simulink model "conSys_3robots_1_vR2014a"  (Simulink 8.3)
settings: Solver=ode3  StartTime=0.0  StopTime=200  FixedStep=Ts  RelTol=1e-3
values from neighbouring files (symbols this model uses):
  ck = double(max(abs([par.q0_r1;par.q0_r2] - [par.q0r_r1;par.q0r_r2]))*20/7000 + 6)    [startUp_conSys_2robots_1_vGPU_vR2014a.m]    (also in startUp_conSys_2robots_1_vR2014a.m = max(abs([par.q0_r1;par.q0_r2] - [par.q0r_r1;par.q0r_r2]))*20; startUp_conSys_2robots_2_vR2014a.m = max(abs([par.q0_r1;par.q0_r2] - [par.q0r_r1;par.q0r_r2]))*20; startUp_conSys_2robots_3_vR2014a.m = max(abs([par.q0_r1;par.q0_r2] - [par.q0r_r1;par.q0r_r2]))*20; startUp_conSys_2robots_4_vR2014a.m = max(abs([par.q0_r1;par.q0_r2] - [par.q0r_r1;par.q0r_r2]))*20)
  d0t = dt*ht    (= 0.328)    [startUp_conSys_2robots_1_vGPU_vR2014a.m]    (also in startUp_conSys_2robots_1_vR2014a.m; startUp_conSys_2robots_2_vR2014a.m; startUp_conSys_2robots_3_vR2014a.m; startUp_conSys_2robots_4_vR2014a.m)
  dt = rt*ht    (= 16.4)    [startUp_conSys_2robots_1_vGPU_vR2014a.m]    (also in startUp_conSys_2robots_1_vR2014a.m; startUp_conSys_2robots_2_vR2014a.m; startUp_conSys_2robots_3_vR2014a.m; startUp_conSys_2robots_4_vR2014a.m)
  dx1r_0 = dxc_0 + sin(thc_0)*dd_0 + d_0*cos(thc_0)*dthc_0    [startUp_conSys_2robots_1_vGPU_vR2014a.m]    (also in startUp_conSys_2robots_1_vR2014a.m; startUp_conSys_2robots_2_vR2014a.m; startUp_conSys_2robots_3_vR2014a.m; startUp_conSys_2robots_4_vR2014a.m)
  dx2r_0 = dxc_0 - sin(thc_0)*dd_0 - d_0*cos(thc_0)*dthc_0    [startUp_conSys_2robots_1_vGPU_vR2014a.m]    (also in startUp_conSys_2robots_1_vR2014a.m; startUp_conSys_2robots_2_vR2014a.m; startUp_conSys_2robots_3_vR2014a.m; startUp_conSys_2robots_4_vR2014a.m)
  dy1r_0 = dyc_0 + cos(thc_0)*dd_0 - d_0*sin(thc_0)*dthc_0    [startUp_conSys_2robots_1_vGPU_vR2014a.m]    (also in startUp_conSys_2robots_1_vR2014a.m; startUp_conSys_2robots_2_vR2014a.m; startUp_conSys_2robots_3_vR2014a.m; startUp_conSys_2robots_4_vR2014a.m)
  dy2r_0 = dyc_0 - cos(thc_0)*dd_0 + d_0*sin(thc_0)*dthc_0    [startUp_conSys_2robots_1_vGPU_vR2014a.m]    (also in startUp_conSys_2robots_1_vR2014a.m; startUp_conSys_2robots_2_vR2014a.m; startUp_conSys_2robots_3_vR2014a.m; startUp_conSys_2robots_4_vR2014a.m)
  ht = .02    (= 0.02)    [startUp_conSys_2robots_1_vGPU_vR2014a.m]    (also in startUp_conSys_2robots_1_vR2014a.m; startUp_conSys_2robots_2_vR2014a.m; startUp_conSys_2robots_3_vR2014a.m; startUp_conSys_2robots_4_vR2014a.m)
  rt = 820    [startUp_conSys_2robots_1_vGPU_vR2014a.m]    (also in startUp_conSys_2robots_1_vR2014a.m; startUp_conSys_2robots_2_vR2014a.m; startUp_conSys_2robots_3_vR2014a.m; startUp_conSys_2robots_4_vR2014a.m)
  TD = ss(Atd,Btd,Ctd,Dtd,Ts)    [startUp_conSys_2robots_1_vGPU_vR2014a.m]    (also in startUp_conSys_2robots_1_vR2014a.m; startUp_conSys_2robots_2_vR2014a.m; startUp_conSys_2robots_3_vR2014a.m; startUp_conSys_2robots_4_vR2014a.m)
  Ts = 1/200    (= 0.005)    [startUp_conSys_2robots_1_vGPU_vR2014a.m]    (also in startUp_conSys_2robots_1_vR2014a.m = 0.0125; startUp_conSys_2robots_2_vR2014a.m = 0.01; startUp_conSys_2robots_3_vR2014a.m; startUp_conSys_2robots_4_vR2014a.m)
undefined symbols (not defined in the file or in its folder): Beta_Correction_1b, Beta_Correction_2b, Beta_Correction_3b, Beta_Correction_4b, DiscIntNeverNeededParam, dth1r_0, dth2r_0, dth3r_0, dx3r_0, dy3r_0, par, th1r_0, th2r_0, th3r_0, x1r_0, x2r_0, x3r_0, y1r_0, y2r_0, y3r_0
undefined symbols (not defined in the file): ADAMS_cwd, ADAMS_exec, ADAMS_host, ADAMS_init, ADAMS_inputs, ADAMS_outputs, ADAMS_prefix, ADAMS_static, ADAMS_sysdir
libraries: simulink x26, cstblocks x11
(part 1 of 3)
settings Model: Creator=baqumau  LastModifiedBy=Mauro
settings DataIOCC: SignalLoggingSaveFormat=Dataset
settings DebuggingCC: UnderspecifiedInitializationDetection=Simplified  StateNameClashWarn=none
settings GRTTargetCC: CombineOutputUpdateFcns=on  GRTInterface=off

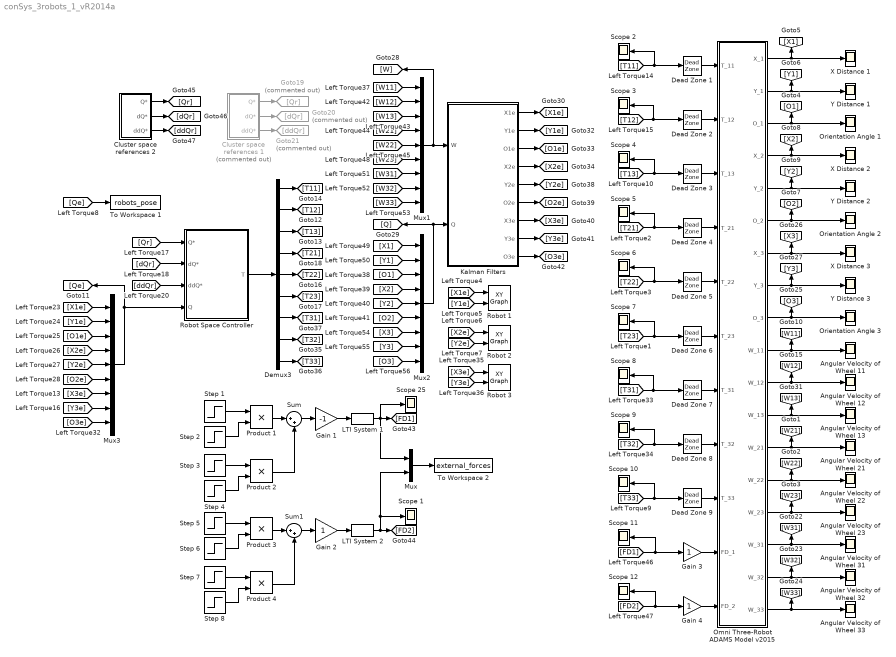
== system conSys_3robots_1_vR2014a ==
  Angular Velocity of Wheel {11..13,21..23,31..33} (9 alike) : Scope
      Angular Velocity of Wheel 11 settings: YMin=-1  YMax=20  SaveName=ScopeData3
      Angular Velocity of Wheel 12 settings: YMin=-1  YMax=1  SaveName=ScopeData2
      Angular Velocity of Wheel 13 settings: YMin=-1  YMax=1  SaveName=ScopeData9
      Angular Velocity of Wheel 21 settings: YMin=-1  YMax=20  SaveName=ScopeData6
      Angular Velocity of Wheel 22 settings: YMin=-1  YMax=1  SaveName=ScopeData10
      Angular Velocity of Wheel 23 settings: YMin=-1  YMax=1  SaveName=ScopeData11
      Angular Velocity of Wheel 31 settings: YMin=-1  YMax=20  SaveName=ScopeData109
      Angular Velocity of Wheel 32 settings: YMin=-1  YMax=1  SaveName=ScopeData110
      Angular Velocity of Wheel 33 settings: YMin=-1  YMax=1  SaveName=ScopeData111
  Cluster space references 1 : Subsystem  Commented=on
  Cluster space references 2 : Subsystem
  Dead Zone {1..9} (9 alike) : DeadZone  LowerValue=-25  UpperValue=25  SaturateOnIntegerOverflow=on
  Demux3 : Demux  Outputs=9
  Gain 1 : Gain  Gain=-1
  Gain 2 : Gain
  Gain 3 : Gain
  Gain 4 : Gain
  Goto19 : Goto  Commented=on  GotoTag=Qr
  Goto20 : Goto  Commented=on  GotoTag=dQr
  Goto21 : Goto  Commented=on  GotoTag=ddQr
  Kalman Filters : Subsystem
  LTI System 1 : cstblocks/LTI System  sys=Fz  IC=[]
  LTI System 2 : cstblocks/LTI System  sys=Fz  IC=[]
  Mux : Mux  Inputs=2
  Mux1 : Mux  Inputs=9
  Mux2 : Mux  Inputs=9
  Mux3 : Mux  Inputs=9
  Omni Three-Robot ADAMS Model v2015 : Subsystem
  Orientation Angle 1 : Scope
      settings: YMin=-3  YMax=3
  Orientation Angle 2 : Scope
      settings: YMin=-3  YMax=3  SaveName=ScopeData12
  Orientation Angle 3 : Scope
      settings: YMin=-3  YMax=3  SaveName=ScopeData112
  Product {1..4} (4 alike) : Product
  Robot 1 : simulink/Sinks/XY Graph  xmin=0  xmax=20000  ymin=0  ymax=20000  st=-1
  Robot 2 : simulink/Sinks/XY Graph  xmin=0  xmax=20000  ymin=0  ymax=20000  st=-1
  Robot 3 : simulink/Sinks/XY Graph  xmin=0  xmax=20000  ymin=0  ymax=20000  st=-1
  Robot Space Controller : Subsystem
  Scope {1..12,25} (13 alike) : Scope
      Scope 1 settings: YMin=-1  YMax=1  SaveName=ScopeData113
      Scope 10 settings: YMin=-6  YMax=6  SaveName=ScopeData124
      Scope 11 settings: YMin=-6  YMax=6  SaveName=ScopeData125
      Scope 12 settings: YMin=-6  YMax=6  SaveName=ScopeData126
      Scope 2 settings: YMin=-6  YMax=6  SaveName=ScopeData114
      Scope 25 settings: YMin=-1  YMax=1  SaveName=ScopeData108
      Scope 3 settings: YMin=-6  YMax=6  SaveName=ScopeData115
      Scope 4 settings: YMin=-6  YMax=6  SaveName=ScopeData116
      Scope 5 settings: YMin=-6  YMax=6  SaveName=ScopeData117
      Scope 6 settings: YMin=-6  YMax=6  SaveName=ScopeData120
      Scope 7 settings: YMin=-6  YMax=6  SaveName=ScopeData121
      Scope 8 settings: YMin=-6  YMax=6  SaveName=ScopeData122
      Scope 9 settings: YMin=-6  YMax=6  SaveName=ScopeData123
  Step 1 : Step  Time=60  SampleTime=0
  Step 2 : Step  Time=100  Before=1  After=0  SampleTime=0
  Step 3 : Step  Time=130  After=-1  SampleTime=0
  Step 4 : Step  Time=170  Before=1  After=0  SampleTime=0
  Step 5 : Step  Time=80  SampleTime=0
  Step 6 : Step  Time=110  Before=1  After=0  SampleTime=0
  Step 7 : Step  Time=120  After=-1  SampleTime=0
  Step 8 : Step  Time=180  Before=1  After=0  SampleTime=0
  Sum : Sum  Inputs=|++
  Sum1 : Sum  Inputs=|++
  To Workspace 1 : ToWorkspace  VariableName=robots_pose  SaveFormat=Structure With Time  SampleTime=-1
  To Workspace 2 : ToWorkspace  VariableName=external_forces  SaveFormat=Structure With Time  SampleTime=-1
  X Distance 1 : Scope
      settings: YMin=0  YMax=10000  SaveName=ScopeData4
  X Distance 2 : Scope
      settings: YMin=0  YMax=10000  SaveName=ScopeData16
  X Distance 3 : Scope
      settings: YMin=0  YMax=10000  SaveName=ScopeData118
  Y Distance 1 : Scope
      settings: YMin=0  YMax=10000
  Y Distance 2 : Scope
      settings: YMin=0  YMax=10000  SaveName=ScopeData17
  Y Distance 3 : Scope
      settings: YMin=3000  YMax=3050  SaveName=ScopeData119
  wires:
  Omni Three-Robot ADAMS Model v2015/1(X_1) -> X Distance 1/1, [X1]
  Omni Three-Robot ADAMS Model v2015/2(Y_1) -> [Y1], Y Distance 1/1
  Omni Three-Robot ADAMS Model v2015/3(O_1) -> [O1], Orientation Angle 1/1
  Omni Three-Robot ADAMS Model v2015/10(W_11) -> [W11], Angular Velocity of Wheel 11/1
  Omni Three-Robot ADAMS Model v2015/11(W_12) -> [W12], Angular Velocity of Wheel 12/1
  Omni Three-Robot ADAMS Model v2015/12(W_13) -> Angular Velocity of Wheel 13/1, [W13]
  Omni Three-Robot ADAMS Model v2015/4(X_2) -> X Distance 2/1, [X2]
  Omni Three-Robot ADAMS Model v2015/5(Y_2) -> Y Distance 2/1, [Y2]
  Omni Three-Robot ADAMS Model v2015/6(O_2) -> Orientation Angle 2/1, [O2]
  Omni Three-Robot ADAMS Model v2015/13(W_21) -> Angular Velocity of Wheel 21/1, [W21]
  Omni Three-Robot ADAMS Model v2015/14(W_22) -> Angular Velocity of Wheel 22/1, [W22]
  Omni Three-Robot ADAMS Model v2015/15(W_23) -> [W23], Angular Velocity of Wheel 23/1
  [X1e] -> Robot 1/1
  [Y1e] -> Robot 1/2
  [X2e] -> Robot 2/1
  [Y2e] -> Robot 2/2
  [O1e] -> Mux3/3
  [X2e] -> Mux3/4
  [Y2e] -> Mux3/5
  [O2e] -> Mux3/6
  [X1e] -> Mux3/1
  [Y1e] -> Mux3/2
  [Qr] -> Robot Space Controller/1(Q*)
  [dQr] -> Robot Space Controller/2(dQ*)
  Mux3/1 -> Robot Space Controller/4(Q), [Qe]
  Robot Space Controller/1(T) -> Demux3/1
  Demux3/1 -> [T11]
  Demux3/2 -> [T12]
  Demux3/3 -> [T13]
  Demux3/4 -> [T21]
  Demux3/5 -> [T22]
  Demux3/6 -> [T23]
  [ddQr] -> Robot Space Controller/3(ddQ*)
  Omni Three-Robot ADAMS Model v2015/7(X_3) -> [X3], X Distance 3/1
  Omni Three-Robot ADAMS Model v2015/8(Y_3) -> [Y3], Y Distance 3/1
  Omni Three-Robot ADAMS Model v2015/9(O_3) -> [O3], Orientation Angle 3/1
  Omni Three-Robot ADAMS Model v2015/16(W_31) -> [W31], Angular Velocity of Wheel 31/1
  Omni Three-Robot ADAMS Model v2015/17(W_32) -> [W32], Angular Velocity of Wheel 32/1
  Omni Three-Robot ADAMS Model v2015/18(W_33) -> Angular Velocity of Wheel 33/1, [W33]
  [X3e] -> Robot 3/1
  [Y3e] -> Robot 3/2
  Cluster space references 1/1(Q*) -> Goto19/1
  Cluster space references 1/2(dQ*) -> Goto20/1
  Cluster space references 1/3(ddQ*) -> Goto21/1
  [X3e] -> Mux3/7
  [Y3e] -> Mux3/8
  [O3e] -> Mux3/9
  Demux3/7 -> [T31]
  Demux3/8 -> [T32]
  Demux3/9 -> [T33]
  [FD2] -> Gain 4/1, Scope 12/1
  [FD1] -> Gain 3/1, Scope 11/1
  [T13] -> Dead Zone 3/1, Scope 4/1
  [T22] -> Dead Zone 5/1, Scope 6/1
  [T31] -> Dead Zone 7/1, Scope 8/1
  [T33] -> Dead Zone 9/1, Scope 10/1
  [T23] -> Dead Zone 6/1, Scope 7/1
  [T12] -> Dead Zone 2/1, Scope 3/1
  [T11] -> Dead Zone 1/1, Scope 2/1
  [T32] -> Dead Zone 8/1, Scope 9/1
  [T21] -> Dead Zone 4/1, Scope 5/1
  [W13] -> Mux1/3
  [W21] -> Mux1/4
  [W22] -> Mux1/5
  [W23] -> Mux1/6
  [W11] -> Mux1/1
  [W12] -> Mux1/2
  Mux1/1 -> [W], Kalman Filters/1(W)
  [O1] -> Mux2/3
  [X2] -> Mux2/4
  [Y2] -> Mux2/5
  [O2] -> Mux2/6
  [X1] -> Mux2/1
  [Y1] -> Mux2/2
  Mux2/1 -> Kalman Filters/2(Q), [Q]
  Kalman Filters/1(X1e) -> [X1e]
  Kalman Filters/2(Y1e) -> [Y1e]
  Kalman Filters/3(O1e) -> [O1e]
  Kalman Filters/4(X2e) -> [X2e]
  Kalman Filters/5(Y2e) -> [Y2e]
  Kalman Filters/6(O2e) -> [O2e]
  [W31] -> Mux1/7
  [W32] -> Mux1/8
  [W33] -> Mux1/9
  [X3] -> Mux2/7
  [Y3] -> Mux2/8
  [O3] -> Mux2/9
  Kalman Filters/7(X3e) -> [X3e]
  Kalman Filters/8(Y3e) -> [Y3e]
  Kalman Filters/9(O3e) -> [O3e]
  [Qe] -> To Workspace 1/1
  Step 1/1 -> Product 1/1
  Step 2/1 -> Product 1/2
  Step 3/1 -> Product 2/1
  Step 4/1 -> Product 2/2
  Product 1/1 -> Sum/1
  Product 2/1 -> Sum/2
  Sum/1 -> Gain 1/1
  Gain 1/1 -> LTI System 1/1
  Step 5/1 -> Product 3/1
  Step 6/1 -> Product 3/2
  Step 7/1 -> Product 4/1
  Step 8/1 -> Product 4/2
  Product 3/1 -> Sum1/1
  Product 4/1 -> Sum1/2
  Sum1/1 -> Gain 2/1
  LTI System 2/1 -> [FD2], Mux/2, Scope 1/1
  Gain 2/1 -> LTI System 2/1
  LTI System 1/1 -> Mux/1, Scope 25/1, [FD1]
  Mux/1 -> To Workspace 2/1
  Cluster space references 2/1(Q*) -> [Qr]
  Cluster space references 2/2(dQ*) -> [dQr]
  Cluster space references 2/3(ddQ*) -> [ddQr]
  Dead Zone 1/1 -> Omni Three-Robot ADAMS Model v2015/1(T_11)
  Dead Zone 2/1 -> Omni Three-Robot ADAMS Model v2015/2(T_12)
  Dead Zone 3/1 -> Omni Three-Robot ADAMS Model v2015/3(T_13)
  Dead Zone 4/1 -> Omni Three-Robot ADAMS Model v2015/4(T_21)
  Dead Zone 5/1 -> Omni Three-Robot ADAMS Model v2015/5(T_22)
  Dead Zone 6/1 -> Omni Three-Robot ADAMS Model v2015/6(T_23)
  Dead Zone 7/1 -> Omni Three-Robot ADAMS Model v2015/7(T_31)
  Dead Zone 8/1 -> Omni Three-Robot ADAMS Model v2015/8(T_32)
  Dead Zone 9/1 -> Omni Three-Robot ADAMS Model v2015/9(T_33)
  Gain 3/1 -> Omni Three-Robot ADAMS Model v2015/10(FD_1)
  Gain 4/1 -> Omni Three-Robot ADAMS Model v2015/11(FD_2)

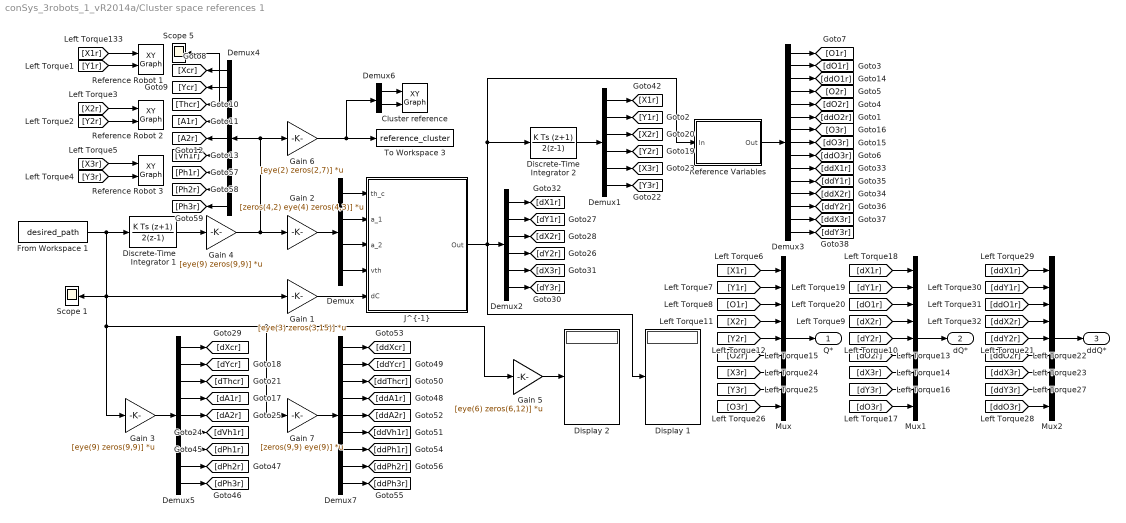
== system conSys_3robots_1_vR2014a/Cluster space references 1 ==
  Cluster reference : simulink/Sinks/XY Graph  xmin=0  xmax=20000  ymin=0  ymax=20000  st=-1
  Demux : Demux
  Demux1 : Demux  Outputs=6
  Demux2 : Demux  Outputs=6
  Demux3 : Demux  Outputs=15
  Demux4 : Demux  Outputs=9
  Demux5 : Demux  Outputs=9
  Demux6 : Demux  Outputs=2
  Demux7 : Demux  Outputs=9
  Discrete-Time Integrator 1 : DiscreteIntegrator  IntegratorMethod=Integration: Trapezoidal  InitialCondition=par.x0_c_ref  SampleTime=Ts  ICPrevOutput=DiscIntNeverNeededParam  ICPrevScaledInput=DiscIntNeverNeededParam
  Discrete-Time Integrator 2 : DiscreteIntegrator  IntegratorMethod=Integration: Trapezoidal  InitialCondition=[x1r_0 y1r_0 x2r_0 y2r_0 x3r_0 y3r_0]'  SampleTime=Ts  ICPrevOutput=DiscIntNeverNeededParam  ICPrevScaledInput=DiscIntNeverNeededParam
  Display 1 : Display
  Display 2 : Display
  From Workspace 1 : FromWorkspace  VariableName=desired_path  SampleTime=Ts  OutputAfterFinalValue=Holding final value
  Gain 1 : Gain  Gain=[eye(3) zeros(3,15)]  Multiplication=Matrix(K*u)
  Gain 2 : Gain  Gain=[zeros(4,2) eye(4) zeros(4,3)]  Multiplication=Matrix(K*u)
  Gain 3 : Gain  Gain=[eye(9) zeros(9,9)]  Multiplication=Matrix(K*u)
  Gain 4 : Gain  Gain=[eye(9) zeros(9,9)]  Multiplication=Matrix(K*u)
  Gain 5 : Gain  Gain=[eye(6) zeros(6,12)]  Multiplication=Matrix(K*u)
  Gain 6 : Gain  Gain=[eye(2) zeros(2,7)]  Multiplication=Matrix(K*u)
  Gain 7 : Gain  Gain=[zeros(9,9) eye(9)]  Multiplication=Matrix(K*u)
  "J^{-1}" : Subsystem
  Mux : Mux  Inputs=9
  Mux1 : Mux  Inputs=9
  Mux2 : Mux  Inputs=9
  Reference Robot 1 : simulink/Sinks/XY Graph  xmin=0  xmax=20000  ymin=0  ymax=20000  st=-1
  Reference Robot 2 : simulink/Sinks/XY Graph  xmin=0  xmax=20000  ymin=0  ymax=20000  st=-1
  Reference Robot 3 : simulink/Sinks/XY Graph  xmin=0  xmax=20000  ymin=0  ymax=20000  st=-1
  Reference Variables : Subsystem
  Scope 1 : Scope
      settings: ShowLegends=on  YMin=-500  YMax=500  SaveName=ScopeData32
  Scope 5 : Scope
      settings: ShowLegends=on  YMin=-500  YMax=500  SaveName=ScopeData100
  To Workspace 3 : ToWorkspace  VariableName=reference_cluster  SaveFormat=Structure With Time  SampleTime=-1
  Q* : Outport
  dQ* : Outport  Port=2
  ddQ* : Outport  Port=3
  wires:
  From Workspace 1/1 -> Scope 1/1, Gain 3/1, Gain 7/1, Gain 5/1, Gain 1/1, Discrete-Time Integrator 1/1
  Discrete-Time Integrator 1/1 -> Gain 4/1
  "J^{-1}"/1(Out) -> Display 1/1, Demux2/1, Reference Variables/1(In), Discrete-Time Integrator 2/1
  Discrete-Time Integrator 2/1 -> Demux1/1
  Demux1/1 -> [X1r]
  Demux1/2 -> [Y1r]
  [X1r] -> Reference Robot 1/1
  [Y1r] -> Reference Robot 1/2
  [X2r] -> Reference Robot 2/1
  [Y2r] -> Reference Robot 2/2
  [X3r] -> Reference Robot 3/1
  [Y3r] -> Reference Robot 3/2
  Demux2/1 -> [dX1r]
  Demux2/2 -> [dY1r]
  Demux2/5 -> [dX3r]
  Demux2/6 -> [dY3r]
  Gain 6/1 -> To Workspace 3/1, Demux6/1
  Demux/2 -> "J^{-1}"/2(a_1)
  Demux/3 -> "J^{-1}"/3(a_2)
  Demux/4 -> "J^{-1}"/4(vth)
  Demux/1 -> "J^{-1}"/1(th_c)
  Gain 1/1 -> "J^{-1}"/5(dC)
  Demux2/3 -> [dX2r]
  Demux2/4 -> [dY2r]
  Demux1/3 -> [X2r]
  Demux1/4 -> [Y2r]
  Demux1/5 -> [X3r]
  Demux1/6 -> [Y3r]
  Reference Variables/1(Out) -> Demux3/1
  Demux3/1 -> [O1r]
  Demux3/2 -> [dO1r]
  Gain 2/1 -> Demux/1
  [X2r] -> Mux/4
  [O1r] -> Mux/3
  [Y1r] -> Mux/2
  [Y2r] -> Mux/5
  [X1r] -> Mux/1
  [O2r] -> Mux/6
  Mux/1 -> Q*/1
  Mux1/1 -> dQ*/1
  Demux4/1 -> [Xcr]
  Demux4/2 -> [Ycr]
  Demux4/3 -> Scope 5/1, [Thcr]
  Demux4/4 -> [A1r]
  Demux4/5 -> [A2r]
  Demux4/6 -> [Vh1r]
  [Y3r] -> Mux/8
  [X3r] -> Mux/7
  [O3r] -> Mux/9
  Demux5/1 -> [dXcr]
  Demux5/2 -> [dYcr]
  Demux5/3 -> [dThcr]
  Demux5/4 -> [dA1r]
  Demux5/5 -> [dA2r]
  Demux5/6 -> [dVh1r]
  Demux6/2 -> Cluster reference/2
  Demux6/1 -> Cluster reference/1
  Gain 3/1 -> Demux5/1
  Gain 4/1 -> Demux4/1, Gain 6/1, Gain 2/1
  Gain 5/1 -> Display 2/1
  Demux5/7 -> [dPh1r]
  Demux5/8 -> [dPh2r]
  Demux5/9 -> [dPh3r]
  Demux7/1 -> [ddXcr]
  Demux7/2 -> [ddYcr]
  Demux7/3 -> [ddThcr]
  Demux7/4 -> [ddA1r]
  Demux7/5 -> [ddA2r]
  Demux7/6 -> [ddVh1r]
  Gain 7/1 -> Demux7/1
  Demux7/7 -> [ddPh1r]
  Demux7/8 -> [ddPh2r]
  Demux7/9 -> [ddPh3r]
  Demux4/7 -> [Ph1r]
  Demux4/8 -> [Ph2r]
  Demux4/9 -> [Ph3r]
  Mux2/1 -> ddQ*/1
  [ddX2r] -> Mux2/4
  [ddO1r] -> Mux2/3
  [ddY1r] -> Mux2/2
  [ddY2r] -> Mux2/5
  [ddX1r] -> Mux2/1
  [ddO2r] -> Mux2/6
  [ddY3r] -> Mux2/8
  [ddX3r] -> Mux2/7
  [ddO3r] -> Mux2/9
  [dX2r] -> Mux1/4
  [dO1r] -> Mux1/3
  [dY1r] -> Mux1/2
  [dY2r] -> Mux1/5
  [dX1r] -> Mux1/1
  [dO2r] -> Mux1/6
  [dY3r] -> Mux1/8
  [dX3r] -> Mux1/7
  [dO3r] -> Mux1/9
  Demux3/3 -> [ddO1r]
  Demux3/4 -> [O2r]
  Demux3/5 -> [dO2r]
  Demux3/6 -> [ddO2r]
  Demux3/7 -> [O3r]
  Demux3/8 -> [dO3r]
  Demux3/9 -> [ddO3r]
  Demux3/10 -> [ddX1r]
  Demux3/11 -> [ddY1r]
  Demux3/12 -> [ddX2r]
  Demux3/13 -> [ddY2r]
  Demux3/14 -> [ddX3r]
  Demux3/15 -> [ddY3r]

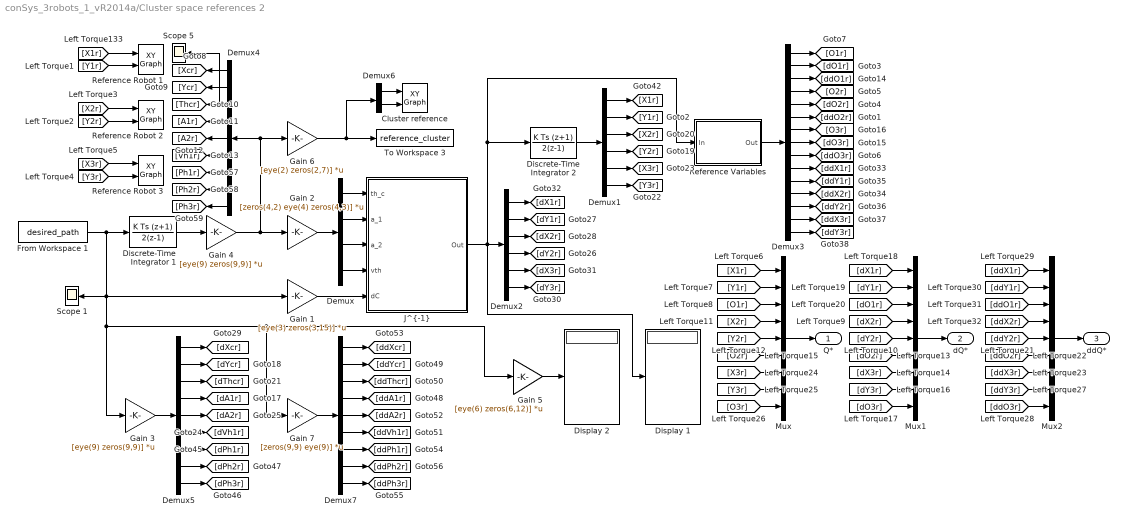
== system conSys_3robots_1_vR2014a/Cluster space references 2 ==
  Cluster reference : simulink/Sinks/XY Graph  xmin=0  xmax=20000  ymin=0  ymax=20000  st=-1
  Demux : Demux
  Demux1 : Demux  Outputs=6
  Demux2 : Demux  Outputs=6
  Demux3 : Demux  Outputs=15
  Demux4 : Demux  Outputs=9
  Demux5 : Demux  Outputs=9
  Demux6 : Demux  Outputs=2
  Demux7 : Demux  Outputs=9
  Discrete-Time Integrator 1 : DiscreteIntegrator  IntegratorMethod=Integration: Trapezoidal  InitialCondition=par.x0_c_ref  SampleTime=Ts  ICPrevOutput=DiscIntNeverNeededParam  ICPrevScaledInput=DiscIntNeverNeededParam
  Discrete-Time Integrator 2 : DiscreteIntegrator  IntegratorMethod=Integration: Trapezoidal  InitialCondition=[x1r_0 y1r_0 x2r_0 y2r_0 x3r_0 y3r_0]'  SampleTime=Ts  ICPrevOutput=DiscIntNeverNeededParam  ICPrevScaledInput=DiscIntNeverNeededParam
  Display 1 : Display
  Display 2 : Display
  From Workspace 1 : FromWorkspace  VariableName=desired_path  SampleTime=Ts  OutputAfterFinalValue=Holding final value
  Gain 1 : Gain  Gain=[eye(3) zeros(3,15)]  Multiplication=Matrix(K*u)
  Gain 2 : Gain  Gain=[zeros(4,2) eye(4) zeros(4,3)]  Multiplication=Matrix(K*u)
  Gain 3 : Gain  Gain=[eye(9) zeros(9,9)]  Multiplication=Matrix(K*u)
  Gain 4 : Gain  Gain=[eye(9) zeros(9,9)]  Multiplication=Matrix(K*u)
  Gain 5 : Gain  Gain=[eye(6) zeros(6,12)]  Multiplication=Matrix(K*u)
  Gain 6 : Gain  Gain=[eye(2) zeros(2,7)]  Multiplication=Matrix(K*u)
  Gain 7 : Gain  Gain=[zeros(9,9) eye(9)]  Multiplication=Matrix(K*u)
  "J^{-1}" : Subsystem
  Mux : Mux  Inputs=9
  Mux1 : Mux  Inputs=9
  Mux2 : Mux  Inputs=9
  Reference Robot 1 : simulink/Sinks/XY Graph  xmin=0  xmax=20000  ymin=0  ymax=20000  st=-1
  Reference Robot 2 : simulink/Sinks/XY Graph  xmin=0  xmax=20000  ymin=0  ymax=20000  st=-1
  Reference Robot 3 : simulink/Sinks/XY Graph  xmin=0  xmax=20000  ymin=0  ymax=20000  st=-1
  Reference Variables : Subsystem
  Scope 1 : Scope
      settings: ShowLegends=on  YMin=-500  YMax=500  SaveName=ScopeData32
  Scope 5 : Scope
      settings: ShowLegends=on  YMin=-500  YMax=500  SaveName=ScopeData100
  To Workspace 3 : ToWorkspace  VariableName=reference_cluster  SaveFormat=Structure With Time  SampleTime=-1
  Q* : Outport
  dQ* : Outport  Port=2
  ddQ* : Outport  Port=3
  wires:
  Demux3/15 -> [ddY3r]
  Demux3/14 -> [ddX3r]
  Demux3/13 -> [ddY2r]
  Demux3/12 -> [ddX2r]
  Demux3/11 -> [ddY1r]
  Demux3/10 -> [ddX1r]
  Demux3/9 -> [ddO3r]
  Demux3/8 -> [dO3r]
  Demux3/7 -> [O3r]
  Demux3/6 -> [ddO2r]
  Demux3/5 -> [dO2r]
  Demux3/4 -> [O2r]
  Demux3/3 -> [ddO1r]
  [dO3r] -> Mux1/9
  [dX3r] -> Mux1/7
  [dY3r] -> Mux1/8
  [dO2r] -> Mux1/6
  [dX1r] -> Mux1/1
  [dY2r] -> Mux1/5
  [dY1r] -> Mux1/2
  [dO1r] -> Mux1/3
  [dX2r] -> Mux1/4
  [ddO3r] -> Mux2/9
  [ddX3r] -> Mux2/7
  [ddY3r] -> Mux2/8
  [ddO2r] -> Mux2/6
  [ddX1r] -> Mux2/1
  [ddY2r] -> Mux2/5
  [ddY1r] -> Mux2/2
  [ddO1r] -> Mux2/3
  [ddX2r] -> Mux2/4
  Mux2/1 -> ddQ*/1
  Demux4/9 -> [Ph3r]
  Demux4/8 -> [Ph2r]
  Demux4/7 -> [Ph1r]
  Demux7/9 -> [ddPh3r]
  Demux7/8 -> [ddPh2r]
  Demux7/7 -> [ddPh1r]
  Gain 7/1 -> Demux7/1
  Demux7/6 -> [ddVh1r]
  Demux7/5 -> [ddA2r]
  Demux7/4 -> [ddA1r]
  Demux7/3 -> [ddThcr]
  Demux7/2 -> [ddYcr]
  Demux7/1 -> [ddXcr]
  Demux5/9 -> [dPh3r]
  Demux5/8 -> [dPh2r]
  Demux5/7 -> [dPh1r]
  Gain 5/1 -> Display 2/1
  Gain 4/1 -> Gain 2/1, Gain 6/1, Demux4/1
  Gain 3/1 -> Demux5/1
  Demux6/1 -> Cluster reference/1
  Demux6/2 -> Cluster reference/2
  Demux5/6 -> [dVh1r]
  Demux5/5 -> [dA2r]
  Demux5/4 -> [dA1r]
  Demux5/3 -> [dThcr]
  Demux5/2 -> [dYcr]
  Demux5/1 -> [dXcr]
  [O3r] -> Mux/9
  [X3r] -> Mux/7
  [Y3r] -> Mux/8
  Demux4/6 -> [Vh1r]
  Demux4/5 -> [A2r]
  Demux4/4 -> [A1r]
  Demux4/3 -> [Thcr], Scope 5/1
  Demux4/2 -> [Ycr]
  Demux4/1 -> [Xcr]
  Mux1/1 -> dQ*/1
  Mux/1 -> Q*/1
  [O2r] -> Mux/6
  [X1r] -> Mux/1
  [Y2r] -> Mux/5
  [Y1r] -> Mux/2
  [O1r] -> Mux/3
  [X2r] -> Mux/4
  Gain 2/1 -> Demux/1
  Demux3/2 -> [dO1r]
  Demux3/1 -> [O1r]
  Reference Variables/1(Out) -> Demux3/1
  Demux1/6 -> [Y3r]
  Demux1/5 -> [X3r]
  Demux1/4 -> [Y2r]
  Demux1/3 -> [X2r]
  Demux2/4 -> [dY2r]
  Demux2/3 -> [dX2r]
  Gain 1/1 -> "J^{-1}"/5(dC)
  Demux/1 -> "J^{-1}"/1(th_c)
  Demux/4 -> "J^{-1}"/4(vth)
  Demux/3 -> "J^{-1}"/3(a_2)
  Demux/2 -> "J^{-1}"/2(a_1)
  Gain 6/1 -> Demux6/1, To Workspace 3/1
  Demux2/6 -> [dY3r]
  Demux2/5 -> [dX3r]
  Demux2/2 -> [dY1r]
  Demux2/1 -> [dX1r]
  [Y3r] -> Reference Robot 3/2
  [X3r] -> Reference Robot 3/1
  [Y2r] -> Reference Robot 2/2
  [X2r] -> Reference Robot 2/1
  [Y1r] -> Reference Robot 1/2
  [X1r] -> Reference Robot 1/1
  Demux1/2 -> [Y1r]
  Demux1/1 -> [X1r]
  Discrete-Time Integrator 2/1 -> Demux1/1
  "J^{-1}"/1(Out) -> Discrete-Time Integrator 2/1, Reference Variables/1(In), Demux2/1, Display 1/1
  Discrete-Time Integrator 1/1 -> Gain 4/1
  From Workspace 1/1 -> Discrete-Time Integrator 1/1, Gain 1/1, Gain 5/1, Gain 7/1, Gain 3/1, Scope 1/1

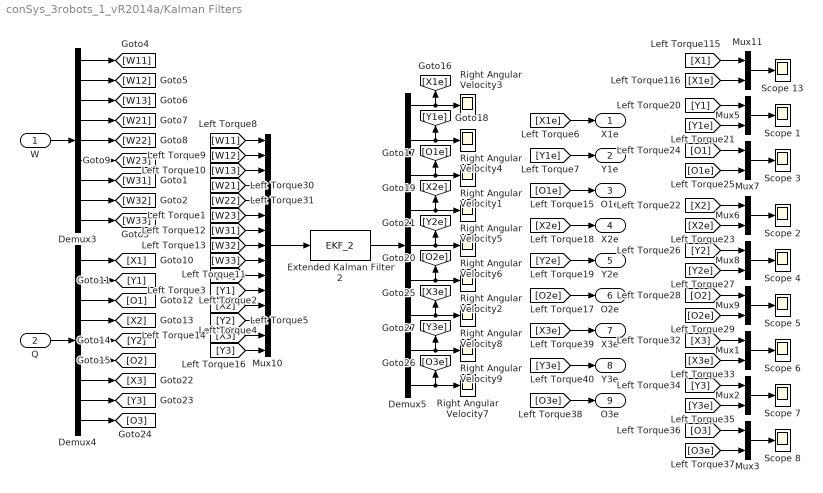
== system conSys_3robots_1_vR2014a/Kalman Filters ==
  W : Inport
  Q : Inport  Port=2
  Demux3 : Demux  Outputs=9
  Demux4 : Demux  Outputs=9
  Demux5 : Demux  Outputs=9
  Extended Kalman Filter 2 : S-Function  FunctionName=EKF_2  Parameters=par  EnableBusSupport=off
  Mux{1..3,5..9,11} (9 alike) : Mux  Inputs=2
  Mux10 : Mux  Inputs=15
  Right Angular Velocity{1..9} (9 alike) : Scope
      Right Angular Velocity1 settings: YMin=-3  YMax=6  SaveName=ScopeData5
      Right Angular Velocity2 settings: YMin=-3  YMax=6  SaveName=ScopeData13
      Right Angular Velocity3 settings: YMin=-10000  YMax=10000  SaveName=ScopeData7
      Right Angular Velocity4 settings: YMin=0  YMax=5000  SaveName=ScopeData8
      Right Angular Velocity5 settings: YMin=-10000  YMax=10000  SaveName=ScopeData14
      Right Angular Velocity6 settings: YMin=0  YMax=5000  SaveName=ScopeData15
      Right Angular Velocity7 settings: YMin=-3  YMax=6  SaveName=ScopeData18
      Right Angular Velocity8 settings: YMin=-10000  YMax=10000  SaveName=ScopeData19
      Right Angular Velocity9 settings: YMin=0  YMax=5000  SaveName=ScopeData20
  Scope {1..8,13} (9 alike) : Scope
      Scope 1 settings: YMin=0  YMax=20000  SaveName=ScopeData29
      Scope 13 settings: YMin=0  YMax=20000  SaveName=ScopeData25
      Scope 2 settings: YMin=-2  YMax=20000  SaveName=ScopeData32
      Scope 3 settings: YMin=-20  YMax=20  SaveName=ScopeData33
      Scope 4 settings: YMin=-2  YMax=20000  SaveName=ScopeData34
      Scope 5 settings: YMin=-20  YMax=20  SaveName=ScopeData35
      Scope 6 settings: YMin=-2  YMax=20000  SaveName=ScopeData21
      Scope 7 settings: YMin=-2  YMax=20000  SaveName=ScopeData23
      Scope 8 settings: YMin=-20  YMax=20  SaveName=ScopeData24
  X1e : Outport
  Y1e : Outport  Port=2
  O1e : Outport  Port=3
  X2e : Outport  Port=4
  Y2e : Outport  Port=5
  O2e : Outport  Port=6
  X3e : Outport  Port=7
  Y3e : Outport  Port=8
  O3e : Outport  Port=9
  wires:
  W/1 -> Demux3/1
  Demux3/1 -> [W11]
  Demux3/2 -> [W12]
  Demux3/3 -> [W13]
  Demux3/4 -> [W21]
  Demux3/5 -> [W22]
  Demux3/6 -> [W23]
  Demux4/1 -> [X1]
  Demux4/2 -> [Y1]
  Demux4/3 -> [O1]
  Demux4/4 -> [X2]
  Demux4/5 -> [Y2]
  Demux4/6 -> [O2]
  Q/1 -> Demux4/1
  [X1e] -> X1e/1
  [Y1e] -> Y1e/1
  [O1e] -> O1e/1
  [X2e] -> X2e/1
  [Y2e] -> Y2e/1
  [O2e] -> O2e/1
  [X1e] -> Mux11/2
  Mux11/1 -> Scope 13/1
  [X1] -> Mux11/1
  [Y1e] -> Mux5/2
  Mux5/1 -> Scope 1/1
  [Y1] -> Mux5/1
  [X2e] -> Mux6/2
  Mux6/1 -> Scope 2/1
  [X2] -> Mux6/1
  [O1e] -> Mux7/2
  Mux7/1 -> Scope 3/1
  [O1] -> Mux7/1
  [Y2e] -> Mux8/2
  Mux8/1 -> Scope 4/1
  [Y2] -> Mux8/1
  [O2e] -> Mux9/2
  Mux9/1 -> Scope 5/1
  [O2] -> Mux9/1
  [W11] -> Mux10/1
  [W12] -> Mux10/2
  [W13] -> Mux10/3
  Mux10/1 -> Extended Kalman Filter 2/1
  Extended Kalman Filter 2/1 -> Demux5/1
  Demux5/2 -> Right Angular Velocity4/1, [Y1e]
  Demux5/3 -> Right Angular Velocity1/1, [O1e]
  Demux5/1 -> Right Angular Velocity3/1, [X1e]
  [W21] -> Mux10/4
  [W22] -> Mux10/5
  Demux5/5 -> [Y2e], Right Angular Velocity6/1
  Demux5/6 -> [O2e], Right Angular Velocity2/1
  Demux5/4 -> [X2e], Right Angular Velocity5/1
  [W23] -> Mux10/6
  Demux3/7 -> [W31]
  Demux3/8 -> [W32]
  Demux3/9 -> [W33]
  Demux4/7 -> [X3]
  Demux4/8 -> [Y3]
  Demux4/9 -> [O3]
  [X2] -> Mux10/12
  [X1] -> Mux10/10
  [Y1] -> Mux10/11
  [Y2] -> Mux10/13
  [X3] -> Mux10/14
  [W31] -> Mux10/7
  [Y3] -> Mux10/15
  [W32] -> Mux10/8
  [W33] -> Mux10/9
  Demux5/8 -> Right Angular Velocity9/1, [Y3e]
  Demux5/9 -> Right Angular Velocity7/1, [O3e]
  Demux5/7 -> Right Angular Velocity8/1, [X3e]
  [X3e] -> Mux1/2
  Mux1/1 -> Scope 6/1
  [X3] -> Mux1/1
  [Y3e] -> Mux2/2
  Mux2/1 -> Scope 7/1
  [Y3] -> Mux2/1
  [O3e] -> Mux3/2
  Mux3/1 -> Scope 8/1
  [O3] -> Mux3/1
  [X3e] -> X3e/1
  [Y3e] -> Y3e/1
  [O3e] -> O3e/1

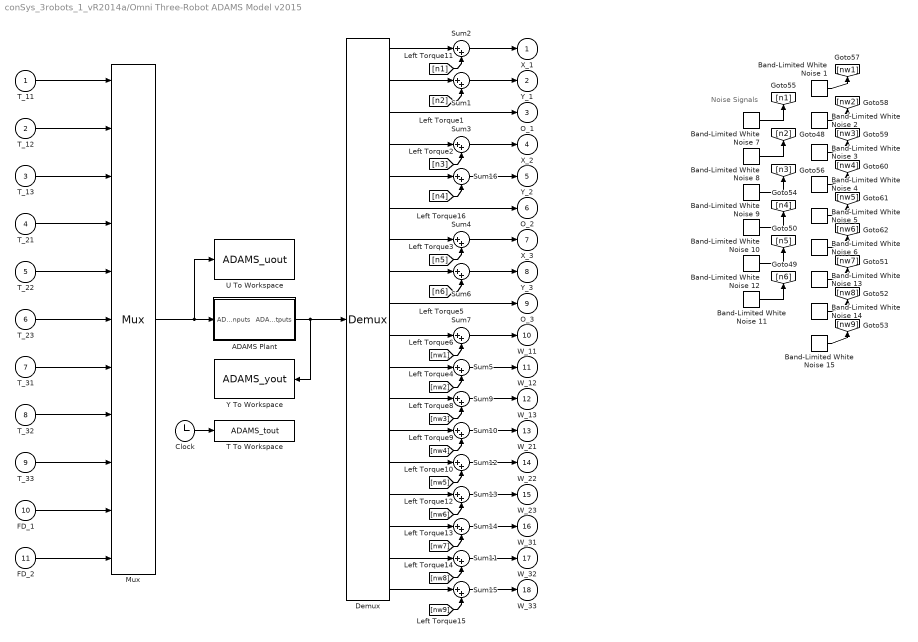
== system conSys_3robots_1_vR2014a/Omni Three-Robot ADAMS Model v2015 ==
  note: Noise Signals
  T_11 : Inport
  T_12 : Inport  Port=2
  T_13 : Inport  Port=3
  T_21 : Inport  Port=4
  T_22 : Inport  Port=5
  T_23 : Inport  Port=6
  T_31 : Inport  Port=7
  T_32 : Inport  Port=8
  T_33 : Inport  Port=9
  FD_1 : Inport  Port=10
  FD_2 : Inport  Port=11
  ADAMS Plant : Subsystem  LoadFcn=|  InitFcn=clear mex  mask(Adams Plant){exevie=ADAMS_sysdir, nam_in=ADAMS_inputs, namout=ADAMS_outputs, nampre=ADAMS_prefix, outfil=ADAMS_prefix, exesol=ADAMS_exec, stat=ADAMS_static, inicmd=[ADAMS_init], exetyp=C++, comtyp=PIPE(DDE), workdir=ADAMS_cwd, ada_host=ADAMS_host, modani=batch, modsim=discrete, dft=no, simulink_lead_cosim=yes, pin_interp_order=0, pout_extrap_order=0, pin_extrap_order=0, pout_interp_order=0, dt_out=Ts, o_rate=1, more=off}
      | %check based on dialog box setting for when setting by popup menu                                             
      | if exist('ADAMS_solver_type')                                                                                 
      |   if strcmp(ADAMS_solver_type,'C++')                                                                          
      |     set_param(gcb,'exetyp','C++');                                                                            
      |   else                                                                                                        
      |     set_param(gcb,'exetyp','Fortran');                                                                        
      |   end                                                                                                         
      | else                                                                                                          
      |   set_param(gcb,'exetyp','C++');                                                                              
      | end                                                                                                           
      | %set the mode if using acar_solver                                                                            
      | %REQUIRED HERE BECAUSE BELOW CAUSES MDLTERMINATE TO BE CALLED 2 TIMES IN MIDDLE OF SIMULATION WHEN SET IN MASK
      |                                                                                                               
      | %enable the direct feedthrough, sim mode, anim mode parameters by default                                     
      |                                                                                                               
      | if exist('set_some_params_states')                                                                            
      |                                                                                                               
      |   set_some_params_states({'dft','modsim','modani'},{'on','on','on'},'MaskEnables',gcb)                        
      |   %turn on direct feedthrough option                                                                          
      |   set_some_params_states({'dft'},{'on'},'MaskVisibilities',gcb)                                               
      |                                                                                                               
      |  end                                                                                                          
      |                                                                                                               
      |                                                                                                               
      | if exist('ADAMS_exec')                                                                                        
      |   if and(strcmp(get_param(gcb,'exesol'),'ADAMS_exec'),strcmp(ADAMS_exec,'acar_solver'))                       
      |     %set the sim mode to discrete -- only supported mode                                                      
      |     set_param(gcb,'modsim','discrete')                                                                        
      |      %turn off direct feedthrough option                                                                      
      |      set_some_params_states({'dft'},{'off'},'MaskVisibilities',gcb)                                           
      |     %set the animation mode to batch -- only supported mode                                                   
      |     set_param(gcb,'modani','batch')                                                                           
      |     %disable the direct feedthrough, sim mode, anim mode parameters                                           
      |     set_some_params_states({'modsim','modani'},{'off','off'},'MaskEnables',gcb)                               
      |   end                                                                                                         
      | end
      mask prompts: exevie "Adams install directory"; nam_in "Adams/View input names"; namout "Adams/View output names"; nampre "Adams model file prefix"; outfil "Output files prefix (opt.: if blank - no output)"; exesol "User executable (opt.: if blank - use standard)"; stat "Initial static simulation flag"; inicmd "Initialization commands"; exetyp "Adams/Solver type"; comtyp "Interprocess option"; workdir "Adams working directory"; ada_host "Adams host"; modani "Animation mode"; modsim "Simulation mode"; dft "Direct feedthrough"; simulink_lead_cosim "Discrete Computational Order - Simulink Leads Adams"; pin_interp_order "Plant input interpolation order"; pout_extrap_order "Plant output extrapolation order"; pin_extrap_order "Plant input extrapolation order"; pout_interp_order "Plant output interpolation order"; dt_out "Communication interval"; o_rate "Number of communications per output step"; more "More parameters"
      mask help: Simulate any Adams plant model either in Adams/Solver form (.adm file) or in Adams/View form (.cmd file)
      settings: OpenFcn=|
      | open_system(gcb,'mask')
      | if not(exist('set_some_params_states'))
      | 
      | warning('The script "set_some_params_states.m" cannot be found in the MATLAB PATH.  Cannot update the ADAMS Plant S-Function parameters.')
      | 
      | warning('Recommended action(optional):  run the Adams/Controls .m file first to help choose the correct settings in the Adams S-Function block.')
      | 
      | end
      mask Help:
      | <html>
      | This S-Function represents the non-linear Adams Plant with the inputs sent to the Adams model <br>
      |  and the outputs generated by the Adams model.  See the Adams/Controls documentation for more <br>
      | information.  This plant uses the following variables:<br>
      | <br>
      | <b>ADAMS_sysdir  :</b> Adams installation directory<br>
      | <b>ADAMS_inputs  :</b> Input variables View names vector<br>
      | <b>ADAMS_outputs :</b> Outputs variables View names vector<br>
      | <b>ADAMS_prefix  : </b>ADAMS model files prefix (.adm, .cmd); also doubles as output files prefix<br>
      | <b>ADAMS_exec :</b> Adams/Solver user library or keyword (e.g., acar_solver)<br>
      | <b>ADAMS_static :</b> yes|no - initial static before Co-simulation(discrete)/Function Evaluation(continuous)<br>
      | <b>ADAMS_init :</b>Initialization commands (i.e., Adams/View or Solver commands, depending on setting for Animation mode)<br>
      | <b>ADAMS_cwd : </b> Current working directory (for TCP/IP)<br>
      | <b>ADAMS_host : </b>Name of Adams server host (for TCP/IP)<br>
      | <b>ADAMS_mode :</b> Linear or non-linear (i.e., co-sim, function eval)<br>
      | <b>ADAMS_solver_type :</b>Fortran or C++ (used to set popup menu when first loaded) <br>
      | 
      | 
      | <br>
      | The following settings can be chosen:<br>
      | <br>
      | <b>Adams/Solver type:</b>  Fortran or C++ (will also set ADAMS_solver_type)<br>
      | <b>Interprocess option:</b> Pipe(DDE) or TCP/IP; TCP/IP can allow different machines run Adams and MATLAB<br>
      | <b>Animation mode:</b> batch (Solver, uses .adm) or interactive (View, uses .cmd)<br>
      | <b>Simulation mode:</b> discrete (Co-simulation) or continuous (Function Evaluation)<br>
      | <b>Discrete Computational Order - Simulink Lead Adams:</b> for discrete mode, chooses if Simulink leads the integration (yes) or lags (no);<br> if set to "no", can remove algebraic loop<br>
      | <b>Plant input interpolation order:</b> 0 = zero-order hold; 1 = linear (discrete mode only, where Simulink leads)<br>
      | <b>Plant output extrapolation order:</b> 0 = zero-order hold;1 = linear(discrete mode only, where Simulink leads)<br>
      | <b>Plant input extrapolation order:</b> 0 = zero-order hold; 1 = linear (discrete mode only, where Adams leads)<br>
      | <b>Plant output interpolation order:</b> 0 = zero-order hold;1 = linear(discrete mode only, where Adams leads)<br>
      | <b>Direct feedthrough:</b> yes|no - yes = Input directly effect output(continuous mode-only)<br>
      | <b>Communication interval:</b> Time step at which Co-simulation exchange information (e.g.,0.005); also controls <br>output for continuous mode (Function Evaluation)<br>
      | <b>Number of communications per output step: </b>Sets Adams output rate (.res, .req, .gra) integer value (default: 1)<br>
      | </html>
      mask Callback exesol:
      | if exist('set_some_params_states')
      | %enable the direct feedthrough, sim mode, anim mode parameters
      | set_some_params_states({'dft','modsim','modani'},{'on','on','on'},'MaskEnables',gcb)
      | %turn on direct feedthrough option
      | set_some_params_states({'dft'},{'on'},'MaskVisibilities',gcb)
      | end
      | 
      | if exist('ADAMS_exec')
      |   if and(strcmp(get_param(gcb,'exesol'),'ADAMS_exec'),strcmp(ADAMS_exec,'acar_solver'))
      |     %set the sim mode to discrete -- only supported mode
      |     %REMOVED:  BELOW CAUSES MDLTERMINATE TO BE CALLED 2 TIMES IN MIDDLE OF SIMULATION
      |     %Now in LoadFcn callback
      |     %set_param(gcb,'modsim','discrete')
      |      %turn off direct feedthrough option
      |     set_some_params_states({'dft'},{'off'},'MaskVisibilities',gcb)
      |     %set the animation mode to batch -- only supported mode
      |     %REMOVED:  BELOW CAUSES MDLTERMINATE TO BE CALLED 2 TIMES IN MIDDLE OF SIMULATION
      |     %Now in LoadFcn callback
      |     %set_param(gcb,'modani','batch')
      |     %disable the direct feedthrough, sim mode, anim mode parameters
      |     set_some_params_states({'modsim','modani'},{'off','off'},'MaskEnables',gcb)
      |   end
      | end
      mask TypeOptions exetyp: Fortran | C++
      mask Callback exetyp:
      | if strcmp(get_param(gcb,'exetyp'),'C++')
      |     ADAMS_solver_type='C++';
      | else
      |     ADAMS_solver_type='Fortran';
      | end
      mask TypeOptions comtyp: PIPE(DDE) | TCP/IP
      mask Callback comtyp:
      | if exist('set_some_params_states')
      | if strcmp(get_param(gcb,'comtyp'),'PIPE(DDE)')
      |     %turn off cwd, host options
      |     set_some_params_states({'ada_host','workdir'},{'off','off'},'MaskVisibilities',gcb)
      | else%if strcmp(get_param(gcb,'modsim'),'TCP/IP')
      |     %turn on cwd, host options
      |     set_some_params_states({'ada_host','workdir'},{'on','on'},'MaskVisibilities',gcb)
      | end
      | end
      mask TypeOptions modani: batch | interactive
      mask TypeOptions modsim: discrete | continuous
      mask Callback modsim:
      | if exist('set_some_params_states')
      | if strcmp(get_param(gcb,'modsim'),'discrete')
      |      %turn off direct feedthrough option
      |     set_some_params_states({'dft'},{'off'},'MaskVisibilities',gcb)
      |     %turn on discrete co-sim type if want to see more
      |     if strcmp(get_param(gcb,'more'),'on')
      |         set_some_params_states({'simulink_lead_cosim'},{'on'},'MaskVisibilities',gcb)
      |     end
      |     if strcmp(get_param(gcb,'simulink_lead_cosim'),'yes')
      |         %turn on interpolation/extrapolation options
      |         set_some_params_states({'pin_interp_order','pout_extrap_order',},{'on','on'},'MaskVisibilities',gcb)
      |     else
      |         set_some_params_states({'pin_extrap_order','pout_interp_order'},{'on','on'},'MaskVisibilities',gcb)
      |     end
      | else%if strcmp(get_param(gcb,'modsim'),'continuous')
      |      %turn off direct feedthrough option
      |     set_some_params_states({'dft'},{'on'},'MaskVisibilities',gcb)
      |     %turn off interpolation/extrapolation options
      |     set_some_params_states({'pin_interp_order','pout_extrap_order','pin_extrap_order','pout_interp_order','simulink_lead_cosim'},{'off','off','off','off','off'},'MaskVisibilities',gcb)
      | end
      | end
      mask TypeOptions dft: no | yes
      mask TypeOptions simulink_lead_cosim: yes | no
      mask Callback simulink_lead_cosim:
      | if exist('set_some_params_states')
      | if (strcmp(get_param(gcb,'simulink_lead_cosim'),'yes') && strcmp(get_param(gcb,'modsim'),'discrete'))
      |      %turn off unused interpolate/extrapolate options
      |     set_some_params_states({'pin_extrap_order','pout_interp_order'},{'off','off'},'MaskVisibilities',gcb)
      |     %turn on used interpolate/extrapolate options
      |     set_some_params_states({'pin_interp_order','pout_extrap_order'},{'on','on'},'MaskVisibilities',gcb)
      | elseif (strcmp(get_param(gcb,'simulink_lead_cosim'),'no') && strcmp(get_param(gcb,'modsim'),'discrete'))
      |     %turn on used interpolate/extrapolate options
      |     set_some_params_states({'pin_extrap_order','pout_interp_order'},{'on','on'},'MaskVisibilities',gcb)
      |      %turn off unused interpolate/extrapolate options
      |     set_some_params_states({'pin_interp_order','pout_extrap_order'},{'off','off'},'MaskVisibilities',gcb)
      | end
      | end
      mask TypeOptions pin_interp_order: 0 | 1
      mask TypeOptions pout_extrap_order: 0 | 1
      mask TypeOptions pin_extrap_order: 0 | 1
      mask TypeOptions pout_interp_order: 0 | 1
      mask Callback more:
      | if exist('set_some_params_states')
      | if (strcmp(get_param(gcb,'more'),'on'))
      |      %turn on infrequently used options
      |     set_some_params_states({'exevie','nam_in','namout','exesol','stat','inicmd'},{'on','on','on','on','on','on'},'MaskVisibilities',gcb)
      |     if strcmp(get_param(gcb,'modsim'),'discrete')
      |         set_some_params_states({'simulink_lead_cosim'},{'on'},'MaskVisibilities',gcb)
      |     end
      | elseif (strcmp(get_param(gcb,'more'),'off'))
      |     %turn off infrequently used options
      |     set_some_params_states({'exevie','nam_in','namout','exesol','stat','inicmd'},{'off','off','off','off','off','off'},'MaskVisibilities',gcb)
      |     if strcmp(get_param(gcb,'modsim'),'discrete')
      |         set_some_params_states({'simulink_lead_cosim'},{'off'},'MaskVisibilities',gcb)
      |     end
      | end
      | end
      mask Display: disp( 'MSC Software' )
  Band-Limited White Noise {1..6,13..15} (9 alike) : simulink/Sources/Band-Limited White Noise  Cov=[0.001]  Ts=Ts  seed=[23341]
  Band-Limited White Noise {7..12} (6 alike) : simulink/Sources/Band-Limited White Noise  Cov=[0.4]  Ts=Ts  seed=[23341]
  Clock : Clock
  Demux : Demux  Outputs=18
  Mux : Mux  Inputs=11
  Sum{1..7,9..16} (15 alike) : Sum  Inputs=|++
  T To Workspace : ToWorkspace  VariableName=ADAMS_tout
      settings: MaxDataPoints=100000
  U To Workspace : ToWorkspace  VariableName=ADAMS_uout
      settings: MaxDataPoints=100000
  Y To Workspace : ToWorkspace  VariableName=ADAMS_yout
      settings: MaxDataPoints=100000
  X_1 : Outport
  Y_1 : Outport  Port=2
  O_1 : Outport  Port=3
  X_2 : Outport  Port=4
  Y_2 : Outport  Port=5
  O_2 : Outport  Port=6
  X_3 : Outport  Port=7
  Y_3 : Outport  Port=8
  O_3 : Outport  Port=9
  W_11 : Outport  Port=10
  W_12 : Outport  Port=11
  W_13 : Outport  Port=12
  W_21 : Outport  Port=13
  W_22 : Outport  Port=14
  W_23 : Outport  Port=15
  W_31 : Outport  Port=16
  W_32 : Outport  Port=17
  W_33 : Outport  Port=18
  wires:
  FD_2/1 -> Mux/11
  FD_1/1 -> Mux/10
  T_33/1 -> Mux/9
  T_32/1 -> Mux/8
  T_31/1 -> Mux/7
  T_23/1 -> Mux/6
  T_22/1 -> Mux/5
  T_21/1 -> Mux/4
  T_13/1 -> Mux/3
  T_12/1 -> Mux/2
  T_11/1 -> Mux/1
  ADAMS Plant/1(ADAMS outputs) -> Y To Workspace/1, Demux/1
  Mux/1 -> U To Workspace/1, ADAMS Plant/1(ADAMS inputs)
  Clock/1 -> T To Workspace/1
  Band-Limited White Noise 7/1 -> [n1]
  Band-Limited White Noise 8/1 -> [n2]
  Band-Limited White Noise 9/1 -> [n3]
  Band-Limited White Noise 10/1 -> [n4]
  Band-Limited White Noise 1/1 -> [nw1]
  Band-Limited White Noise 2/1 -> [nw2]
  Band-Limited White Noise 3/1 -> [nw3]
  Band-Limited White Noise 4/1 -> [nw4]
  Band-Limited White Noise 5/1 -> [nw5]
  Band-Limited White Noise 6/1 -> [nw6]
  Band-Limited White Noise 12/1 -> [n5]
  Band-Limited White Noise 11/1 -> [n6]
  Band-Limited White Noise 13/1 -> [nw7]
  Band-Limited White Noise 14/1 -> [nw8]
  Band-Limited White Noise 15/1 -> [nw9]
  Demux/1 -> Sum2/1
  Sum2/1 -> X_1/1
  [n1] -> Sum2/2
  Demux/2 -> Sum1/1
  Sum1/1 -> Y_1/1
  [n2] -> Sum1/2
  Demux/4 -> Sum3/1
  Sum3/1 -> X_2/1
  [n3] -> Sum3/2
  Demux/8 -> Sum6/1
  Sum6/1 -> Y_3/1
  [n6] -> Sum6/2
  Demux/10 -> Sum7/1
  [nw1] -> Sum7/2
  Demux/12 -> Sum9/1
  [nw3] -> Sum9/2
  Demux/13 -> Sum10/1
  [nw4] -> Sum10/2
  Demux/14 -> Sum12/1
  [nw5] -> Sum12/2
  Demux/15 -> Sum13/1
  [nw6] -> Sum13/2
  Demux/16 -> Sum14/1
  [nw7] -> Sum14/2
  Demux/17 -> Sum11/1
  [nw8] -> Sum11/2
  Demux/18 -> Sum15/1
  [nw9] -> Sum15/2
  Sum7/1 -> W_11/1
  Sum9/1 -> W_13/1
  Sum10/1 -> W_21/1
  Sum12/1 -> W_22/1
  Sum13/1 -> W_23/1
  Sum14/1 -> W_31/1
  Sum11/1 -> W_32/1
  Sum15/1 -> W_33/1
  ? -> ?
  Demux/5 -> Sum16/1
  Sum16/1 -> Y_2/1
  [n4] -> Sum16/2
  Demux/7 -> Sum4/1
  Sum4/1 -> X_3/1
  [n5] -> Sum4/2
  ? -> ?
  ? -> ?
  Demux/11 -> Sum5/1
  [nw2] -> Sum5/2
  Sum5/1 -> W_12/1
  Demux/3 -> O_1/1
  Demux/6 -> O_2/1
  Demux/9 -> O_3/1
